simulink model "ZynqBF_2tx_fpga"  (R2018b)
settings: Solver=FixedStepDiscrete  StartTime=0.0  StopTime=10.0  FixedStep=(1/420e3)/128  RelTol=1e-3
undefined symbols (not defined in the file): a, b, c, gs1_i, gs1_q, gs2_i, gs2_q, gs_length
libraries: hdlsllib x65, simulink x41
(part 3 of 4)

== system ZynqBF_2tx_fpga/channel_estimator/peakdetect_ch1/correlator1/sum_elements_i ==
  din : Inport  Partition=on  PartitionDimension=1  PartitionWidth=8  PartitionOffset=0
  start : Inport  Port=2
  Add : Sum  OutDataTypeStr=fixdt(1,32,16)
  Compare To Constant1 : simulink/Logic and Bit Operations/Compare To Constant  relop===  const=7  OutDataTypeStr=boolean
  Compare To Constant2 : simulink/Logic and Bit Operations/Compare To Constant  relop===  const=1  OutDataTypeStr=boolean
  Constant : Constant  Value=0  OutDataTypeStr=fixdt(1,32,16)  SampleTime=-1
  Constant1 : Constant  Value=0  OutDataTypeStr=fixdt(1,16,15)  SampleTime=-1
  Data Type Conversion : DataTypeConversion  OutDataTypeStr=uint8
  Delay1 : Delay  DelayLength=1
  For Each : ForEach  DisableCoverage=on  IndexMode=One-based
  HDL Counter : hdlsllib/Sources/HDL Counter  CountType=Free running  CountInit=0  CountStep=1  CountMax=64  CountFromType=Initial value  CountFrom=0  CountResetPort=on  CountLoadPort=off  CountEnbPort=on  CountDirPort=off  CountDataType=Unsigned  CountWordLen=3  CountFracLen=0  CountSampTime=1
      settings: SourceProductBaseCode=HD
  HDL Counter1 : hdlsllib/Sources/HDL Counter  CountType=Free running  CountInit=0  CountStep=1  CountMax=64  CountFromType=Initial value  CountFrom=0  CountResetPort=off  CountLoadPort=off  CountEnbPort=on  CountDirPort=off  CountDataType=Unsigned  CountWordLen=1  CountFracLen=0  CountSampTime=1
      settings: SourceProductBaseCode=HD
  Logical Operator : Logic  Operator=OR  IconShape=distinctive  AllPortsSameDT=off  OutDataTypeStr=boolean
  Selector : Selector  IndexMode=Zero-based  InputPortWidth=8  IndexOptions=Starting index (port)  Indices=[1 3]  OutputSizes=1
  Switch : Switch  Criteria=u2 ~= 0
  Switch1 : Switch  Criteria=u2 ~= 0
  dout : Outport  ConcatenationDimension=1
  vout : Outport  Port=2  ConcatenationDimension=1
  wires:
  start/1 -> Logical Operator/1, Switch/2, HDL Counter/1
  Add/1 -> Delay1/1, dout/1
  Compare To Constant2/1 -> Switch1/2, HDL Counter/2
  Compare To Constant1/1 -> Logical Operator/2, vout/1
  Delay1/1 -> Switch/3
  Switch/1 -> Add/2
  Constant/1 -> Switch/1
  Switch1/1 -> Add/1
  Constant1/1 -> Switch1/3
  HDL Counter1/1 -> Compare To Constant2/1
  Selector/1 -> Switch1/1
  din/1 -> Selector/1
  Data Type Conversion/1 -> Selector/2
  Logical Operator/1 -> HDL Counter1/1
  HDL Counter/1 -> Compare To Constant1/1, Data Type Conversion/1

== system ZynqBF_2tx_fpga/channel_estimator/peakdetect_ch1/correlator1/sum_elements_q ==
  din : Inport  Partition=on  PartitionDimension=1  PartitionWidth=8  PartitionOffset=0
  start : Inport  Port=2
  Add : Sum  OutDataTypeStr=fixdt(1,32,16)
  Compare To Constant1 : simulink/Logic and Bit Operations/Compare To Constant  relop===  const=7  OutDataTypeStr=boolean
  Compare To Constant2 : simulink/Logic and Bit Operations/Compare To Constant  relop===  const=1  OutDataTypeStr=boolean
  Constant : Constant  Value=0  OutDataTypeStr=fixdt(1,32,16)  SampleTime=-1
  Constant1 : Constant  Value=0  OutDataTypeStr=fixdt(1,16,15)  SampleTime=-1
  Data Type Conversion : DataTypeConversion  OutDataTypeStr=uint8
  Delay1 : Delay  DelayLength=1
  For Each : ForEach  DisableCoverage=on  IndexMode=One-based
  HDL Counter : hdlsllib/Sources/HDL Counter  CountType=Free running  CountInit=0  CountStep=1  CountMax=64  CountFromType=Initial value  CountFrom=0  CountResetPort=on  CountLoadPort=off  CountEnbPort=on  CountDirPort=off  CountDataType=Unsigned  CountWordLen=3  CountFracLen=0  CountSampTime=1
      settings: SourceProductBaseCode=HD
  HDL Counter1 : hdlsllib/Sources/HDL Counter  CountType=Free running  CountInit=0  CountStep=1  CountMax=64  CountFromType=Initial value  CountFrom=0  CountResetPort=off  CountLoadPort=off  CountEnbPort=on  CountDirPort=off  CountDataType=Unsigned  CountWordLen=1  CountFracLen=0  CountSampTime=1
      settings: SourceProductBaseCode=HD
  Logical Operator : Logic  Operator=OR  IconShape=distinctive  AllPortsSameDT=off  OutDataTypeStr=boolean
  Selector : Selector  IndexMode=Zero-based  InputPortWidth=8  IndexOptions=Starting index (port)  Indices=[1 3]  OutputSizes=1
  Switch : Switch  Criteria=u2 ~= 0
  Switch1 : Switch  Criteria=u2 ~= 0
  dout : Outport  ConcatenationDimension=1
  vout : Outport  Port=2  ConcatenationDimension=1
  wires:
  start/1 -> Logical Operator/1, Switch/2, HDL Counter/1
  Add/1 -> Delay1/1, dout/1
  Compare To Constant2/1 -> Switch1/2, HDL Counter/2
  Compare To Constant1/1 -> Logical Operator/2, vout/1
  Delay1/1 -> Switch/3
  Switch/1 -> Add/2
  Constant/1 -> Switch/1
  Switch1/1 -> Add/1
  Constant1/1 -> Switch1/3
  HDL Counter1/1 -> Compare To Constant2/1
  Selector/1 -> Switch1/1
  din/1 -> Selector/1
  Data Type Conversion/1 -> Selector/2
  Logical Operator/1 -> HDL Counter1/1
  HDL Counter/1 -> Compare To Constant1/1, Data Type Conversion/1

== system ZynqBF_2tx_fpga/channel_estimator/peakdetect_ch2/correlator2/correlation_config ==
  rst : Inport
  vin : Inport  Port=2
  Bit Slice : hdlsllib/Logic and Bit Operations/Bit Slice  lidx=14  ridx=6
  Delay{1..2,4..5} (4 alike) : Delay  DelayLength=1
  Delay6 : Delay  DelayLength=3
  correlation_count : hdlsllib/Sources/HDL Counter  CountType=Free running  CountInit=2^15 - 1  CountStep=1  CountMax=25  CountFromType=Initial value  CountFrom=2^15 - 1  CountResetPort=on  CountLoadPort=off  CountEnbPort=on  CountDirPort=off  CountDataType=Unsigned  CountWordLen=15  CountFracLen=0  CountSampTime=1
      settings: SourceProductBaseCode=HD
  shift_count : hdlsllib/Sources/HDL Counter  CountType=Free running  CountInit=63  CountStep=1  CountMax=1  CountFromType=Initial value  CountFrom=63  CountResetPort=on  CountLoadPort=off  CountEnbPort=on  CountDirPort=off  CountDataType=Unsigned  CountWordLen=6  CountFracLen=0  CountSampTime=1
      settings: SourceProductBaseCode=HD
  addr : Outport
  shift : Outport  Port=2
  vout : Outport  Port=3
  wires:
  Delay6/1 -> vout/1
  shift_count/1 -> Delay5/1
  Delay5/1 -> shift/1
  Delay4/1 -> correlation_count/1, shift_count/1
  Delay2/1 -> addr/1
  Delay1/1 -> correlation_count/2, shift_count/2, Delay6/1
  rst/1 -> Delay4/1
  Bit Slice/1 -> Delay2/1
  vin/1 -> Delay1/1
  correlation_count/1 -> Bit Slice/1

== system ZynqBF_2tx_fpga/channel_estimator/peakdetect_ch2/correlator2/correlator_en ==
  valid : Inport
  done : Inport  Port=2
  addri : Inport  Port=3
  Compare To Constant : simulink/Logic and Bit Operations/Compare To Constant  relop===  const=1  OutDataTypeStr=boolean
  Delay1 : Delay  DelayLength=1
  Delay2 : Delay  DelayLength=1
  Delay3 : Delay  DelayLength=1
  Sum : Sum  Inputs=|++
  corr_addr : hdlsllib/Sources/HDL Counter  CountType=Count limited  CountInit=0  CountStep=1  CountMax=63  CountFromType=Initial value  CountFrom=0  CountResetPort=on  CountLoadPort=off  CountEnbPort=on  CountDirPort=off  CountDataType=Unsigned  CountWordLen=6  CountFracLen=0  CountSampTime=1
      settings: SourceProductBaseCode=HD
  corr_state : hdlsllib/Sources/HDL Counter  CountType=Count limited  CountInit=0  CountStep=1  CountMax=1  CountFromType=Initial value  CountFrom=0  CountResetPort=on  CountLoadPort=off  CountEnbPort=on  CountDirPort=off  CountDataType=Unsigned  CountWordLen=6  CountFracLen=0  CountSampTime=1
      settings: SourceProductBaseCode=HD
  start : Outport
  en : Outport  Port=2
  gs_addr : Outport  Port=3
  rx_addr : Outport  Port=4
  wires:
  addri/1 -> Sum/2
  Sum/1 -> rx_addr/1
  corr_addr/1 -> Sum/1, gs_addr/1
  Delay3/1 -> start/1
  Delay2/1 -> en/1, corr_addr/2
  Delay1/1 -> Delay3/1, corr_state/2
  done/1 -> corr_state/1
  Compare To Constant/1 -> Delay2/1
  corr_state/1 -> Compare To Constant/1
  valid/1 -> Delay1/1, corr_addr/1

== system ZynqBF_2tx_fpga/channel_estimator/peakdetect_ch2/correlator2/correlator_i ==
  rx : Inport  Partition=on  PartitionDimension=1  PartitionWidth=1  PartitionOffset=0
  gs : Inport  Port=2  Partition=on  PartitionDimension=1  PartitionWidth=1  PartitionOffset=0
  start : Inport  Port=3
  vin : Inport  Port=4
  Compare To Constant1 : simulink/Logic and Bit Operations/Compare To Constant  relop===  const=63  OutDataTypeStr=boolean
  Constant : Constant  Value=0  OutDataTypeStr=fixdt(1,32,16)  SampleTime=-1
  Constant1 : Constant  Value=0  OutDataTypeStr=fixdt(1,16,15)  SampleTime=-1
  Delay1 : Delay  DelayLength=1
  For Each : ForEach  DisableCoverage=on  IndexMode=One-based
  HDL Counter : hdlsllib/Sources/HDL Counter  CountType=Free running  CountInit=0  CountStep=1  CountMax=64  CountFromType=Initial value  CountFrom=0  CountResetPort=on  CountLoadPort=off  CountEnbPort=on  CountDirPort=off  CountDataType=Unsigned  CountWordLen=7  CountFracLen=0  CountSampTime=1
      settings: SourceProductBaseCode=HD
  Multiply-Add : hdlsllib/HDL Operations/Multiply-Add  Function=c+(a.*b)  datatype=fixdt(1,32,16)  DoSatur=off  FMA=off
      settings: SourceProductName=HDL Coder  SourceProductBaseCode=HD
  Switch : Switch  Criteria=u2 ~= 0
  Switch1 : Switch  Criteria=u2 ~= 0
  Switch2 : Switch  Criteria=u2 ~= 0
  correlator_mac : hdlsllib/HDL Operations/Multiply-Accumulate  Commented=on  opMode=Streaming - using Start and End ports  initValueSetting=Dialog  initValue=0  initValueSetting2=Dialog  initValue2=0  initValueSetting3=Dialog  initValue3=0  num_samples=2  RndMeth2=Floor  RndMeth3=Floor  datatype2=Inherit: Inherit via back propagation  datatype3=Inherit: Inherit via back propagation  validOut=off  endInandOut=on  startOut=off  countOut=on  dim=-1  DoSatur=off  parallel=off
      settings: SourceProductName=HDL Coder  SourceProductBaseCode=HD
  dout : Outport  ConcatenationDimension=1
  vout : Outport  Port=2  ConcatenationDimension=1
  wires:
  Constant1/1 -> Switch2/3, Switch1/3
  Switch2/1 -> Multiply-Add/2
  Switch1/1 -> Multiply-Add/1
  Constant/1 -> Switch/1
  Switch/1 -> Multiply-Add/3
  Delay1/1 -> Switch/3
  gs/1 -> Switch2/1
  Compare To Constant1/1 -> vout/1
  HDL Counter/1 -> Compare To Constant1/1
  vin/1 -> HDL Counter/2, Switch2/2, Switch1/2
  Multiply-Add/1 -> dout/1, Delay1/1
  start/1 -> HDL Counter/1, Switch/2
  rx/1 -> Switch1/1

== system ZynqBF_2tx_fpga/channel_estimator/peakdetect_ch2/correlator2/correlator_q ==
  rx : Inport  Partition=on  PartitionDimension=1  PartitionWidth=1  PartitionOffset=0
  gs : Inport  Port=2  Partition=on  PartitionDimension=1  PartitionWidth=1  PartitionOffset=0
  start : Inport  Port=3
  vin : Inport  Port=4
  Compare To Constant1 : simulink/Logic and Bit Operations/Compare To Constant  relop===  const=63  OutDataTypeStr=boolean
  Constant : Constant  Value=0  OutDataTypeStr=fixdt(1,32,16)  SampleTime=-1
  Constant1 : Constant  Value=0  OutDataTypeStr=fixdt(1,16,15)  SampleTime=-1
  Delay1 : Delay  DelayLength=1
  For Each : ForEach  DisableCoverage=on  IndexMode=One-based
  HDL Counter : hdlsllib/Sources/HDL Counter  CountType=Free running  CountInit=0  CountStep=1  CountMax=64  CountFromType=Initial value  CountFrom=0  CountResetPort=on  CountLoadPort=off  CountEnbPort=on  CountDirPort=off  CountDataType=Unsigned  CountWordLen=7  CountFracLen=0  CountSampTime=1
      settings: SourceProductBaseCode=HD
  Multiply-Add : hdlsllib/HDL Operations/Multiply-Add  Function=c+(a.*b)  datatype=fixdt(1,32,16)  DoSatur=off  FMA=off
      settings: SourceProductName=HDL Coder  SourceProductBaseCode=HD
  Switch : Switch  Criteria=u2 ~= 0
  Switch1 : Switch  Criteria=u2 ~= 0
  Switch2 : Switch  Criteria=u2 ~= 0
  correlator_mac : hdlsllib/HDL Operations/Multiply-Accumulate  Commented=on  opMode=Streaming - using Start and End ports  initValueSetting=Dialog  initValue=0  initValueSetting2=Dialog  initValue2=0  initValueSetting3=Dialog  initValue3=0  num_samples=2  RndMeth2=Floor  RndMeth3=Floor  datatype2=Inherit: Inherit via back propagation  datatype3=Inherit: Inherit via back propagation  validOut=off  endInandOut=on  startOut=off  countOut=on  dim=-1  DoSatur=off  parallel=off
      settings: SourceProductName=HDL Coder  SourceProductBaseCode=HD
  dout : Outport  ConcatenationDimension=1
  vout : Outport  Port=2  ConcatenationDimension=1
  wires:
  Constant1/1 -> Switch2/3, Switch1/3
  Switch2/1 -> Multiply-Add/2
  Switch1/1 -> Multiply-Add/1
  Constant/1 -> Switch/1
  Switch/1 -> Multiply-Add/3
  Delay1/1 -> Switch/3
  gs/1 -> Switch2/1
  Compare To Constant1/1 -> vout/1
  HDL Counter/1 -> Compare To Constant1/1
  vin/1 -> HDL Counter/2, Switch2/2, Switch1/2
  Multiply-Add/1 -> dout/1, Delay1/1
  start/1 -> HDL Counter/1, Switch/2
  rx/1 -> Switch1/1

== system ZynqBF_2tx_fpga/channel_estimator/peakdetect_ch2/correlator2/data_in ==
  rst : Inport
  valid : Inport  Port=2
  Bit Rotate : hdlsllib/Logic and Bit Operations/Bit Rotate  mode=Rotate Left  N=1
      settings: SourceProductName=HDL Coder  SourceProductBaseCode=HD
  Compare To Constant : simulink/Logic and Bit Operations/Compare To Constant  relop===  const=63  OutDataTypeStr=boolean
  Constant1 : Constant  Value=0  OutDataTypeStr=fixdt(0,64,0)  SampleTime=-1
  Delay{,2..4,6} (5 alike) : Delay  DelayLength=1
  Delay1 : Delay  DelayLength=1  InitialCondition=(2^63)
  Delay5 : Delay  DelayLength=3
  Logical Operator : Logic  IconShape=distinctive  AllPortsSameDT=off  OutDataTypeStr=boolean
  Switch1 : Switch  Criteria=u2 ~= 0
  Switch2 : Switch  Criteria=u2 ~= 0
  addr_counter : hdlsllib/Sources/HDL Counter  CountType=Count limited  CountInit=63  CountStep=1  CountMax=511  CountFromType=Initial value  CountFrom=63  CountResetPort=on  CountLoadPort=off  CountEnbPort=on  CountDirPort=off  CountDataType=Unsigned  CountWordLen=9  CountFracLen=0  CountSampTime=1
      settings: SourceProductBaseCode=HD
  ram_counter : hdlsllib/Sources/HDL Counter  CountType=Free running  CountInit=63  CountStep=1  CountMax=63  CountFromType=Initial value  CountFrom=63  CountResetPort=on  CountLoadPort=off  CountEnbPort=on  CountDirPort=off  CountDataType=Unsigned  CountWordLen=6  CountFracLen=0  CountSampTime=1
      settings: SourceProductBaseCode=HD
  addr : Outport
  we : Outport  Port=2
  wires:
  Delay5/1 -> addr/1
  Delay6/1 -> Delay/1, Switch1/2
  Delay4/1 -> addr_counter/1, ram_counter/1  "rst"
  Delay3/1 -> ram_counter/2, Logical Operator/2, Delay6/1
  Delay2/1 -> we/1
  Switch2/1 -> Delay2/1
  Delay/1 -> Switch2/2
  Constant1/1 -> Switch2/3
  Bit Rotate/1 -> Switch1/1
  Switch1/1 -> Switch2/1, Delay1/1
  Delay1/1 -> Bit Rotate/1, Switch1/3
  Compare To Constant/1 -> Logical Operator/1
  Logical Operator/1 -> addr_counter/2
  rst/1 -> Delay4/1
  ram_counter/1 -> Compare To Constant/1
  valid/1 -> Delay3/1
  addr_counter/1 -> Delay5/1

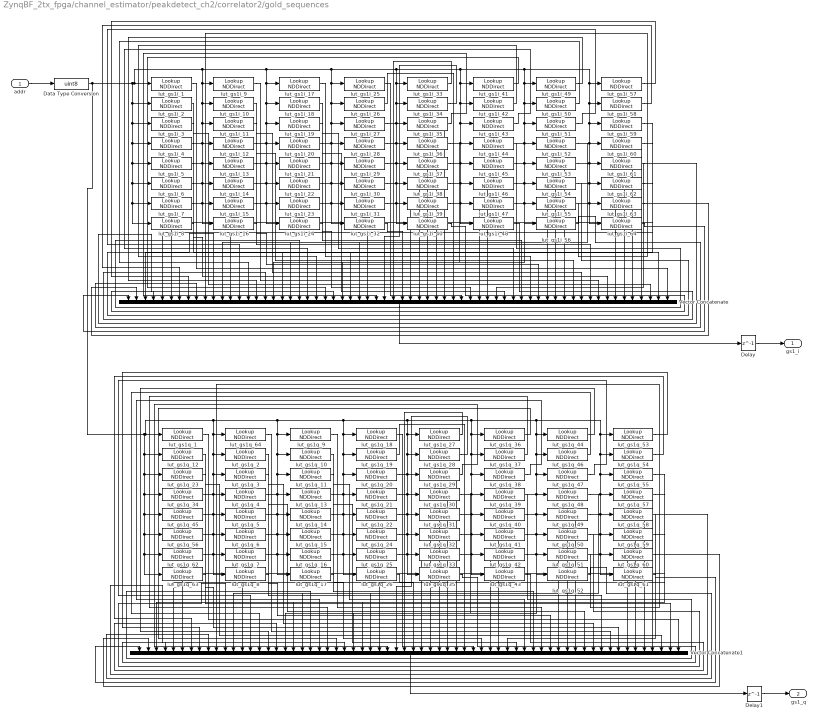
== system ZynqBF_2tx_fpga/channel_estimator/peakdetect_ch2/correlator2/gold_sequences ==
  addr : Inport
  Data Type Conversion : DataTypeConversion  OutDataTypeStr=uint8
  Delay : Delay  DelayLength=1
  Delay1 : Delay  DelayLength=1
  Vector Concatenate : Concatenate  NumInputs=64
  Vector Concatenate1 : Concatenate  NumInputs=64
  lut_gs1i_1 : LookupNDDirect  NumberOfTableDimensions=1  Table=gs2_i_f(1:64:end)  DiagnosticForOutOfRangeInput=Error  TableDataTypeStr=fixdt(1,16,15)
  lut_gs1i_10 : LookupNDDirect  NumberOfTableDimensions=1  Table=gs2_i_f(10:64:end)  DiagnosticForOutOfRangeInput=Error  TableDataTypeStr=fixdt(1,16,15)
  lut_gs1i_11 : LookupNDDirect  NumberOfTableDimensions=1  Table=gs2_i_f(11:64:end)  DiagnosticForOutOfRangeInput=Error  TableDataTypeStr=fixdt(1,16,15)
  lut_gs1i_12 : LookupNDDirect  NumberOfTableDimensions=1  Table=gs2_i_f(12:64:end)  DiagnosticForOutOfRangeInput=Error  TableDataTypeStr=fixdt(1,16,15)
  lut_gs1i_13 : LookupNDDirect  NumberOfTableDimensions=1  Table=gs2_i_f(13:64:end)  DiagnosticForOutOfRangeInput=Error  TableDataTypeStr=fixdt(1,16,15)
  lut_gs1i_14 : LookupNDDirect  NumberOfTableDimensions=1  Table=gs2_i_f(14:64:end)  DiagnosticForOutOfRangeInput=Error  TableDataTypeStr=fixdt(1,16,15)
  lut_gs1i_15 : LookupNDDirect  NumberOfTableDimensions=1  Table=gs2_i_f(15:64:end)  DiagnosticForOutOfRangeInput=Error  TableDataTypeStr=fixdt(1,16,15)
  lut_gs1i_16 : LookupNDDirect  NumberOfTableDimensions=1  Table=gs2_i_f(16:64:end)  DiagnosticForOutOfRangeInput=Error  TableDataTypeStr=fixdt(1,16,15)
  lut_gs1i_17 : LookupNDDirect  NumberOfTableDimensions=1  Table=gs2_i_f(17:64:end)  DiagnosticForOutOfRangeInput=Error  TableDataTypeStr=fixdt(1,16,15)
  lut_gs1i_18 : LookupNDDirect  NumberOfTableDimensions=1  Table=gs2_i_f(18:64:end)  DiagnosticForOutOfRangeInput=Error  TableDataTypeStr=fixdt(1,16,15)
  lut_gs1i_19 : LookupNDDirect  NumberOfTableDimensions=1  Table=gs2_i_f(19:64:end)  DiagnosticForOutOfRangeInput=Error  TableDataTypeStr=fixdt(1,16,15)
  lut_gs1i_2 : LookupNDDirect  NumberOfTableDimensions=1  Table=gs2_i_f(2:64:end)  DiagnosticForOutOfRangeInput=Error  TableDataTypeStr=fixdt(1,16,15)
  lut_gs1i_20 : LookupNDDirect  NumberOfTableDimensions=1  Table=gs2_i_f(20:64:end)  DiagnosticForOutOfRangeInput=Error  TableDataTypeStr=fixdt(1,16,15)
  lut_gs1i_21 : LookupNDDirect  NumberOfTableDimensions=1  Table=gs2_i_f(21:64:end)  DiagnosticForOutOfRangeInput=Error  TableDataTypeStr=fixdt(1,16,15)
  lut_gs1i_22 : LookupNDDirect  NumberOfTableDimensions=1  Table=gs2_i_f(22:64:end)  DiagnosticForOutOfRangeInput=Error  TableDataTypeStr=fixdt(1,16,15)
  lut_gs1i_23 : LookupNDDirect  NumberOfTableDimensions=1  Table=gs2_i_f(23:64:end)  DiagnosticForOutOfRangeInput=Error  TableDataTypeStr=fixdt(1,16,15)
  lut_gs1i_24 : LookupNDDirect  NumberOfTableDimensions=1  Table=gs2_i_f(24:64:end)  DiagnosticForOutOfRangeInput=Error  TableDataTypeStr=fixdt(1,16,15)
  lut_gs1i_25 : LookupNDDirect  NumberOfTableDimensions=1  Table=gs2_i_f(25:64:end)  DiagnosticForOutOfRangeInput=Error  TableDataTypeStr=fixdt(1,16,15)
  lut_gs1i_26 : LookupNDDirect  NumberOfTableDimensions=1  Table=gs2_i_f(26:64:end)  DiagnosticForOutOfRangeInput=Error  TableDataTypeStr=fixdt(1,16,15)
  lut_gs1i_27 : LookupNDDirect  NumberOfTableDimensions=1  Table=gs2_i_f(27:64:end)  DiagnosticForOutOfRangeInput=Error  TableDataTypeStr=fixdt(1,16,15)
  lut_gs1i_28 : LookupNDDirect  NumberOfTableDimensions=1  Table=gs2_i_f(28:64:end)  DiagnosticForOutOfRangeInput=Error  TableDataTypeStr=fixdt(1,16,15)
  lut_gs1i_29 : LookupNDDirect  NumberOfTableDimensions=1  Table=gs2_i_f(29:64:end)  DiagnosticForOutOfRangeInput=Error  TableDataTypeStr=fixdt(1,16,15)
  lut_gs1i_3 : LookupNDDirect  NumberOfTableDimensions=1  Table=gs2_i_f(3:64:end)  DiagnosticForOutOfRangeInput=Error  TableDataTypeStr=fixdt(1,16,15)
  lut_gs1i_30 : LookupNDDirect  NumberOfTableDimensions=1  Table=gs2_i_f(30:64:end)  DiagnosticForOutOfRangeInput=Error  TableDataTypeStr=fixdt(1,16,15)
  lut_gs1i_31 : LookupNDDirect  NumberOfTableDimensions=1  Table=gs2_i_f(31:64:end)  DiagnosticForOutOfRangeInput=Error  TableDataTypeStr=fixdt(1,16,15)
  lut_gs1i_32 : LookupNDDirect  NumberOfTableDimensions=1  Table=gs2_i_f(32:64:end)  DiagnosticForOutOfRangeInput=Error  TableDataTypeStr=fixdt(1,16,15)
  lut_gs1i_33 : LookupNDDirect  NumberOfTableDimensions=1  Table=gs2_i_f(33:64:end)  DiagnosticForOutOfRangeInput=Error  TableDataTypeStr=fixdt(1,16,15)
  lut_gs1i_34 : LookupNDDirect  NumberOfTableDimensions=1  Table=gs2_i_f(34:64:end)  DiagnosticForOutOfRangeInput=Error  TableDataTypeStr=fixdt(1,16,15)
  lut_gs1i_35 : LookupNDDirect  NumberOfTableDimensions=1  Table=gs2_i_f(35:64:end)  DiagnosticForOutOfRangeInput=Error  TableDataTypeStr=fixdt(1,16,15)
  lut_gs1i_36 : LookupNDDirect  NumberOfTableDimensions=1  Table=gs2_i_f(36:64:end)  DiagnosticForOutOfRangeInput=Error  TableDataTypeStr=fixdt(1,16,15)
  lut_gs1i_37 : LookupNDDirect  NumberOfTableDimensions=1  Table=gs2_i_f(37:64:end)  DiagnosticForOutOfRangeInput=Error  TableDataTypeStr=fixdt(1,16,15)
  lut_gs1i_38 : LookupNDDirect  NumberOfTableDimensions=1  Table=gs2_i_f(38:64:end)  DiagnosticForOutOfRangeInput=Error  TableDataTypeStr=fixdt(1,16,15)
  lut_gs1i_39 : LookupNDDirect  NumberOfTableDimensions=1  Table=gs2_i_f(39:64:end)  DiagnosticForOutOfRangeInput=Error  TableDataTypeStr=fixdt(1,16,15)
  lut_gs1i_4 : LookupNDDirect  NumberOfTableDimensions=1  Table=gs2_i_f(4:64:end)  DiagnosticForOutOfRangeInput=Error  TableDataTypeStr=fixdt(1,16,15)
  lut_gs1i_40 : LookupNDDirect  NumberOfTableDimensions=1  Table=gs2_i_f(40:64:end)  DiagnosticForOutOfRangeInput=Error  TableDataTypeStr=fixdt(1,16,15)
  lut_gs1i_41 : LookupNDDirect  NumberOfTableDimensions=1  Table=gs2_i_f(41:64:end)  DiagnosticForOutOfRangeInput=Error  TableDataTypeStr=fixdt(1,16,15)
  lut_gs1i_42 : LookupNDDirect  NumberOfTableDimensions=1  Table=gs2_i_f(42:64:end)  DiagnosticForOutOfRangeInput=Error  TableDataTypeStr=fixdt(1,16,15)
  lut_gs1i_43 : LookupNDDirect  NumberOfTableDimensions=1  Table=gs2_i_f(43:64:end)  DiagnosticForOutOfRangeInput=Error  TableDataTypeStr=fixdt(1,16,15)
  lut_gs1i_44 : LookupNDDirect  NumberOfTableDimensions=1  Table=gs2_i_f(44:64:end)  DiagnosticForOutOfRangeInput=Error  TableDataTypeStr=fixdt(1,16,15)
  lut_gs1i_45 : LookupNDDirect  NumberOfTableDimensions=1  Table=gs2_i_f(45:64:end)  DiagnosticForOutOfRangeInput=Error  TableDataTypeStr=fixdt(1,16,15)
  lut_gs1i_46 : LookupNDDirect  NumberOfTableDimensions=1  Table=gs2_i_f(46:64:end)  DiagnosticForOutOfRangeInput=Error  TableDataTypeStr=fixdt(1,16,15)
  lut_gs1i_47 : LookupNDDirect  NumberOfTableDimensions=1  Table=gs2_i_f(47:64:end)  DiagnosticForOutOfRangeInput=Error  TableDataTypeStr=fixdt(1,16,15)
  lut_gs1i_48 : LookupNDDirect  NumberOfTableDimensions=1  Table=gs2_i_f(48:64:end)  DiagnosticForOutOfRangeInput=Error  TableDataTypeStr=fixdt(1,16,15)
  lut_gs1i_49 : LookupNDDirect  NumberOfTableDimensions=1  Table=gs2_i_f(49:64:end)  DiagnosticForOutOfRangeInput=Error  TableDataTypeStr=fixdt(1,16,15)
  lut_gs1i_5 : LookupNDDirect  NumberOfTableDimensions=1  Table=gs2_i_f(5:64:end)  DiagnosticForOutOfRangeInput=Error  TableDataTypeStr=fixdt(1,16,15)
  lut_gs1i_50 : LookupNDDirect  NumberOfTableDimensions=1  Table=gs2_i_f(50:64:end)  DiagnosticForOutOfRangeInput=Error  TableDataTypeStr=fixdt(1,16,15)
  lut_gs1i_51 : LookupNDDirect  NumberOfTableDimensions=1  Table=gs2_i_f(51:64:end)  DiagnosticForOutOfRangeInput=Error  TableDataTypeStr=fixdt(1,16,15)
  lut_gs1i_52 : LookupNDDirect  NumberOfTableDimensions=1  Table=gs2_i_f(52:64:end)  DiagnosticForOutOfRangeInput=Error  TableDataTypeStr=fixdt(1,16,15)
  lut_gs1i_53 : LookupNDDirect  NumberOfTableDimensions=1  Table=gs2_i_f(53:64:end)  DiagnosticForOutOfRangeInput=Error  TableDataTypeStr=fixdt(1,16,15)
  lut_gs1i_54 : LookupNDDirect  NumberOfTableDimensions=1  Table=gs2_i_f(54:64:end)  DiagnosticForOutOfRangeInput=Error  TableDataTypeStr=fixdt(1,16,15)
  lut_gs1i_55 : LookupNDDirect  NumberOfTableDimensions=1  Table=gs2_i_f(55:64:end)  DiagnosticForOutOfRangeInput=Error  TableDataTypeStr=fixdt(1,16,15)
  lut_gs1i_56 : LookupNDDirect  NumberOfTableDimensions=1  Table=gs2_i_f(56:64:end)  DiagnosticForOutOfRangeInput=Error  TableDataTypeStr=fixdt(1,16,15)
  lut_gs1i_57 : LookupNDDirect  NumberOfTableDimensions=1  Table=gs2_i_f(57:64:end)  DiagnosticForOutOfRangeInput=Error  TableDataTypeStr=fixdt(1,16,15)
  lut_gs1i_58 : LookupNDDirect  NumberOfTableDimensions=1  Table=gs2_i_f(58:64:end)  DiagnosticForOutOfRangeInput=Error  TableDataTypeStr=fixdt(1,16,15)
  lut_gs1i_59 : LookupNDDirect  NumberOfTableDimensions=1  Table=gs2_i_f(59:64:end)  DiagnosticForOutOfRangeInput=Error  TableDataTypeStr=fixdt(1,16,15)
  lut_gs1i_6 : LookupNDDirect  NumberOfTableDimensions=1  Table=gs2_i_f(6:64:end)  DiagnosticForOutOfRangeInput=Error  TableDataTypeStr=fixdt(1,16,15)
  lut_gs1i_60 : LookupNDDirect  NumberOfTableDimensions=1  Table=gs2_i_f(60:64:end)  DiagnosticForOutOfRangeInput=Error  TableDataTypeStr=fixdt(1,16,15)
  lut_gs1i_61 : LookupNDDirect  NumberOfTableDimensions=1  Table=gs2_i_f(61:64:end)  DiagnosticForOutOfRangeInput=Error  TableDataTypeStr=fixdt(1,16,15)
  lut_gs1i_62 : LookupNDDirect  NumberOfTableDimensions=1  Table=gs2_i_f(62:64:end)  DiagnosticForOutOfRangeInput=Error  TableDataTypeStr=fixdt(1,16,15)
  lut_gs1i_63 : LookupNDDirect  NumberOfTableDimensions=1  Table=gs2_i_f(63:64:end)  DiagnosticForOutOfRangeInput=Error  TableDataTypeStr=fixdt(1,16,15)
  lut_gs1i_64 : LookupNDDirect  NumberOfTableDimensions=1  Table=gs2_i_f(64:64:end)  DiagnosticForOutOfRangeInput=Error  TableDataTypeStr=fixdt(1,16,15)
  lut_gs1i_7 : LookupNDDirect  NumberOfTableDimensions=1  Table=gs2_i_f(7:64:end)  DiagnosticForOutOfRangeInput=Error  TableDataTypeStr=fixdt(1,16,15)
  lut_gs1i_8 : LookupNDDirect  NumberOfTableDimensions=1  Table=gs2_i_f(8:64:end)  DiagnosticForOutOfRangeInput=Error  TableDataTypeStr=fixdt(1,16,15)
  lut_gs1i_9 : LookupNDDirect  NumberOfTableDimensions=1  Table=gs2_i_f(9:64:end)  DiagnosticForOutOfRangeInput=Error  TableDataTypeStr=fixdt(1,16,15)
  lut_gs1q_1 : LookupNDDirect  NumberOfTableDimensions=1  Table=gs2_q_f(1:64:end)  DiagnosticForOutOfRangeInput=Error  TableDataTypeStr=fixdt(1,16,15)
  lut_gs1q_10 : LookupNDDirect  NumberOfTableDimensions=1  Table=gs2_q_f(18:64:end)  DiagnosticForOutOfRangeInput=Error  TableDataTypeStr=fixdt(1,16,15)
  lut_gs1q_11 : LookupNDDirect  NumberOfTableDimensions=1  Table=gs2_q_f(19:64:end)  DiagnosticForOutOfRangeInput=Error  TableDataTypeStr=fixdt(1,16,15)
  lut_gs1q_12 : LookupNDDirect  NumberOfTableDimensions=1  Table=gs2_q_f(2:64:end)  DiagnosticForOutOfRangeInput=Error  TableDataTypeStr=fixdt(1,16,15)
  lut_gs1q_13 : LookupNDDirect  NumberOfTableDimensions=1  Table=gs2_q_f(20:64:end)  DiagnosticForOutOfRangeInput=Error  TableDataTypeStr=fixdt(1,16,15)
  lut_gs1q_14 : LookupNDDirect  NumberOfTableDimensions=1  Table=gs2_q_f(21:64:end)  DiagnosticForOutOfRangeInput=Error  TableDataTypeStr=fixdt(1,16,15)
  lut_gs1q_15 : LookupNDDirect  NumberOfTableDimensions=1  Table=gs2_q_f(22:64:end)  DiagnosticForOutOfRangeInput=Error  TableDataTypeStr=fixdt(1,16,15)
  lut_gs1q_16 : LookupNDDirect  NumberOfTableDimensions=1  Table=gs2_q_f(23:64:end)  DiagnosticForOutOfRangeInput=Error  TableDataTypeStr=fixdt(1,16,15)
  lut_gs1q_17 : LookupNDDirect  NumberOfTableDimensions=1  Table=gs2_q_f(24:64:end)  DiagnosticForOutOfRangeInput=Error  TableDataTypeStr=fixdt(1,16,15)
  lut_gs1q_18 : LookupNDDirect  NumberOfTableDimensions=1  Table=gs2_q_f(25:64:end)  DiagnosticForOutOfRangeInput=Error  TableDataTypeStr=fixdt(1,16,15)
  lut_gs1q_19 : LookupNDDirect  NumberOfTableDimensions=1  Table=gs2_q_f(26:64:end)  DiagnosticForOutOfRangeInput=Error  TableDataTypeStr=fixdt(1,16,15)
  lut_gs1q_2 : LookupNDDirect  NumberOfTableDimensions=1  Table=gs2_q_f(10:64:end)  DiagnosticForOutOfRangeInput=Error  TableDataTypeStr=fixdt(1,16,15)
  lut_gs1q_20 : LookupNDDirect  NumberOfTableDimensions=1  Table=gs2_q_f(27:64:end)  DiagnosticForOutOfRangeInput=Error  TableDataTypeStr=fixdt(1,16,15)
  lut_gs1q_21 : LookupNDDirect  NumberOfTableDimensions=1  Table=gs2_q_f(28:64:end)  DiagnosticForOutOfRangeInput=Error  TableDataTypeStr=fixdt(1,16,15)
  lut_gs1q_22 : LookupNDDirect  NumberOfTableDimensions=1  Table=gs2_q_f(29:64:end)  DiagnosticForOutOfRangeInput=Error  TableDataTypeStr=fixdt(1,16,15)
  lut_gs1q_23 : LookupNDDirect  NumberOfTableDimensions=1  Table=gs2_q_f(3:64:end)  DiagnosticForOutOfRangeInput=Error  TableDataTypeStr=fixdt(1,16,15)
  lut_gs1q_24 : LookupNDDirect  NumberOfTableDimensions=1  Table=gs2_q_f(30:64:end)  DiagnosticForOutOfRangeInput=Error  TableDataTypeStr=fixdt(1,16,15)
  lut_gs1q_25 : LookupNDDirect  NumberOfTableDimensions=1  Table=gs2_q_f(31:64:end)  DiagnosticForOutOfRangeInput=Error  TableDataTypeStr=fixdt(1,16,15)
  lut_gs1q_26 : LookupNDDirect  NumberOfTableDimensions=1  Table=gs2_q_f(32:64:end)  DiagnosticForOutOfRangeInput=Error  TableDataTypeStr=fixdt(1,16,15)
  lut_gs1q_27 : LookupNDDirect  NumberOfTableDimensions=1  Table=gs2_q_f(33:64:end)  DiagnosticForOutOfRangeInput=Error  TableDataTypeStr=fixdt(1,16,15)
  lut_gs1q_28 : LookupNDDirect  NumberOfTableDimensions=1  Table=gs2_q_f(34:64:end)  DiagnosticForOutOfRangeInput=Error  TableDataTypeStr=fixdt(1,16,15)
  lut_gs1q_29 : LookupNDDirect  NumberOfTableDimensions=1  Table=gs2_q_f(35:64:end)  DiagnosticForOutOfRangeInput=Error  TableDataTypeStr=fixdt(1,16,15)
  lut_gs1q_3 : LookupNDDirect  NumberOfTableDimensions=1  Table=gs2_q_f(11:64:end)  DiagnosticForOutOfRangeInput=Error  TableDataTypeStr=fixdt(1,16,15)
  lut_gs1q_30 : LookupNDDirect  NumberOfTableDimensions=1  Table=gs2_q_f(36:64:end)  DiagnosticForOutOfRangeInput=Error  TableDataTypeStr=fixdt(1,16,15)
  lut_gs1q_31 : LookupNDDirect  NumberOfTableDimensions=1  Table=gs2_q_f(37:64:end)  DiagnosticForOutOfRangeInput=Error  TableDataTypeStr=fixdt(1,16,15)
  lut_gs1q_32 : LookupNDDirect  NumberOfTableDimensions=1  Table=gs2_q_f(38:64:end)  DiagnosticForOutOfRangeInput=Error  TableDataTypeStr=fixdt(1,16,15)
  lut_gs1q_33 : LookupNDDirect  NumberOfTableDimensions=1  Table=gs2_q_f(39:64:end)  DiagnosticForOutOfRangeInput=Error  TableDataTypeStr=fixdt(1,16,15)
  lut_gs1q_34 : LookupNDDirect  NumberOfTableDimensions=1  Table=gs2_q_f(4:64:end)  DiagnosticForOutOfRangeInput=Error  TableDataTypeStr=fixdt(1,16,15)
  lut_gs1q_35 : LookupNDDirect  NumberOfTableDimensions=1  Table=gs2_q_f(40:64:end)  DiagnosticForOutOfRangeInput=Error  TableDataTypeStr=fixdt(1,16,15)
  lut_gs1q_36 : LookupNDDirect  NumberOfTableDimensions=1  Table=gs2_q_f(41:64:end)  DiagnosticForOutOfRangeInput=Error  TableDataTypeStr=fixdt(1,16,15)
  lut_gs1q_37 : LookupNDDirect  NumberOfTableDimensions=1  Table=gs2_q_f(42:64:end)  DiagnosticForOutOfRangeInput=Error  TableDataTypeStr=fixdt(1,16,15)
  lut_gs1q_38 : LookupNDDirect  NumberOfTableDimensions=1  Table=gs2_q_f(43:64:end)  DiagnosticForOutOfRangeInput=Error  TableDataTypeStr=fixdt(1,16,15)
  lut_gs1q_39 : LookupNDDirect  NumberOfTableDimensions=1  Table=gs2_q_f(44:64:end)  DiagnosticForOutOfRangeInput=Error  TableDataTypeStr=fixdt(1,16,15)
  lut_gs1q_4 : LookupNDDirect  NumberOfTableDimensions=1  Table=gs2_q_f(12:64:end)  DiagnosticForOutOfRangeInput=Error  TableDataTypeStr=fixdt(1,16,15)
  lut_gs1q_40 : LookupNDDirect  NumberOfTableDimensions=1  Table=gs2_q_f(45:64:end)  DiagnosticForOutOfRangeInput=Error  TableDataTypeStr=fixdt(1,16,15)
  lut_gs1q_41 : LookupNDDirect  NumberOfTableDimensions=1  Table=gs2_q_f(46:64:end)  DiagnosticForOutOfRangeInput=Error  TableDataTypeStr=fixdt(1,16,15)
  lut_gs1q_42 : LookupNDDirect  NumberOfTableDimensions=1  Table=gs2_q_f(47:64:end)  DiagnosticForOutOfRangeInput=Error  TableDataTypeStr=fixdt(1,16,15)
  lut_gs1q_43 : LookupNDDirect  NumberOfTableDimensions=1  Table=gs2_q_f(48:64:end)  DiagnosticForOutOfRangeInput=Error  TableDataTypeStr=fixdt(1,16,15)
  lut_gs1q_44 : LookupNDDirect  NumberOfTableDimensions=1  Table=gs2_q_f(49:64:end)  DiagnosticForOutOfRangeInput=Error  TableDataTypeStr=fixdt(1,16,15)
  lut_gs1q_45 : LookupNDDirect  NumberOfTableDimensions=1  Table=gs2_q_f(5:64:end)  DiagnosticForOutOfRangeInput=Error  TableDataTypeStr=fixdt(1,16,15)
  lut_gs1q_46 : LookupNDDirect  NumberOfTableDimensions=1  Table=gs2_q_f(50:64:end)  DiagnosticForOutOfRangeInput=Error  TableDataTypeStr=fixdt(1,16,15)
  lut_gs1q_47 : LookupNDDirect  NumberOfTableDimensions=1  Table=gs2_q_f(51:64:end)  DiagnosticForOutOfRangeInput=Error  TableDataTypeStr=fixdt(1,16,15)
  lut_gs1q_48 : LookupNDDirect  NumberOfTableDimensions=1  Table=gs2_q_f(52:64:end)  DiagnosticForOutOfRangeInput=Error  TableDataTypeStr=fixdt(1,16,15)
  lut_gs1q_49 : LookupNDDirect  NumberOfTableDimensions=1  Table=gs2_q_f(53:64:end)  DiagnosticForOutOfRangeInput=Error  TableDataTypeStr=fixdt(1,16,15)
  lut_gs1q_5 : LookupNDDirect  NumberOfTableDimensions=1  Table=gs2_q_f(13:64:end)  DiagnosticForOutOfRangeInput=Error  TableDataTypeStr=fixdt(1,16,15)
  lut_gs1q_50 : LookupNDDirect  NumberOfTableDimensions=1  Table=gs2_q_f(54:64:end)  DiagnosticForOutOfRangeInput=Error  TableDataTypeStr=fixdt(1,16,15)
  lut_gs1q_51 : LookupNDDirect  NumberOfTableDimensions=1  Table=gs2_q_f(55:64:end)  DiagnosticForOutOfRangeInput=Error  TableDataTypeStr=fixdt(1,16,15)
  lut_gs1q_52 : LookupNDDirect  NumberOfTableDimensions=1  Table=gs2_q_f(56:64:end)  DiagnosticForOutOfRangeInput=Error  TableDataTypeStr=fixdt(1,16,15)
  lut_gs1q_53 : LookupNDDirect  NumberOfTableDimensions=1  Table=gs2_q_f(57:64:end)  DiagnosticForOutOfRangeInput=Error  TableDataTypeStr=fixdt(1,16,15)
  lut_gs1q_54 : LookupNDDirect  NumberOfTableDimensions=1  Table=gs2_q_f(58:64:end)  DiagnosticForOutOfRangeInput=Error  TableDataTypeStr=fixdt(1,16,15)
  lut_gs1q_55 : LookupNDDirect  NumberOfTableDimensions=1  Table=gs2_q_f(59:64:end)  DiagnosticForOutOfRangeInput=Error  TableDataTypeStr=fixdt(1,16,15)
  lut_gs1q_56 : LookupNDDirect  NumberOfTableDimensions=1  Table=gs2_q_f(6:64:end)  DiagnosticForOutOfRangeInput=Error  TableDataTypeStr=fixdt(1,16,15)
  lut_gs1q_57 : LookupNDDirect  NumberOfTableDimensions=1  Table=gs2_q_f(60:64:end)  DiagnosticForOutOfRangeInput=Error  TableDataTypeStr=fixdt(1,16,15)
  lut_gs1q_58 : LookupNDDirect  NumberOfTableDimensions=1  Table=gs2_q_f(61:64:end)  DiagnosticForOutOfRangeInput=Error  TableDataTypeStr=fixdt(1,16,15)
  lut_gs1q_59 : LookupNDDirect  NumberOfTableDimensions=1  Table=gs2_q_f(62:64:end)  DiagnosticForOutOfRangeInput=Error  TableDataTypeStr=fixdt(1,16,15)
  lut_gs1q_6 : LookupNDDirect  NumberOfTableDimensions=1  Table=gs2_q_f(14:64:end)  DiagnosticForOutOfRangeInput=Error  TableDataTypeStr=fixdt(1,16,15)
  lut_gs1q_60 : LookupNDDirect  NumberOfTableDimensions=1  Table=gs2_q_f(63:64:end)  DiagnosticForOutOfRangeInput=Error  TableDataTypeStr=fixdt(1,16,15)
  lut_gs1q_61 : LookupNDDirect  NumberOfTableDimensions=1  Table=gs2_q_f(64:64:end)  DiagnosticForOutOfRangeInput=Error  TableDataTypeStr=fixdt(1,16,15)
  lut_gs1q_62 : LookupNDDirect  NumberOfTableDimensions=1  Table=gs2_q_f(7:64:end)  DiagnosticForOutOfRangeInput=Error  TableDataTypeStr=fixdt(1,16,15)
  lut_gs1q_63 : LookupNDDirect  NumberOfTableDimensions=1  Table=gs2_q_f(8:64:end)  DiagnosticForOutOfRangeInput=Error  TableDataTypeStr=fixdt(1,16,15)
  lut_gs1q_64 : LookupNDDirect  NumberOfTableDimensions=1  Table=gs2_q_f(9:64:end)  DiagnosticForOutOfRangeInput=Error  TableDataTypeStr=fixdt(1,16,15)
  lut_gs1q_7 : LookupNDDirect  NumberOfTableDimensions=1  Table=gs2_q_f(15:64:end)  DiagnosticForOutOfRangeInput=Error  TableDataTypeStr=fixdt(1,16,15)
  lut_gs1q_8 : LookupNDDirect  NumberOfTableDimensions=1  Table=gs2_q_f(16:64:end)  DiagnosticForOutOfRangeInput=Error  TableDataTypeStr=fixdt(1,16,15)
  lut_gs1q_9 : LookupNDDirect  NumberOfTableDimensions=1  Table=gs2_q_f(17:64:end)  DiagnosticForOutOfRangeInput=Error  TableDataTypeStr=fixdt(1,16,15)
  gs1_i : Outport
  gs1_q : Outport  Port=2
  wires:
  addr/1 -> Data Type Conversion/1
  Delay/1 -> gs1_i/1
  Delay1/1 -> gs1_q/1
  lut_gs1i_1/1 -> Vector Concatenate/64
  lut_gs1i_2/1 -> Vector Concatenate/63
  lut_gs1i_3/1 -> Vector Concatenate/62
  lut_gs1i_4/1 -> Vector Concatenate/61
  lut_gs1i_5/1 -> Vector Concatenate/60
  lut_gs1i_6/1 -> Vector Concatenate/59
  lut_gs1i_7/1 -> Vector Concatenate/58
  lut_gs1i_8/1 -> Vector Concatenate/57
  lut_gs1i_9/1 -> Vector Concatenate/56
  lut_gs1i_10/1 -> Vector Concatenate/55
  lut_gs1i_11/1 -> Vector Concatenate/54
  lut_gs1i_12/1 -> Vector Concatenate/53
  lut_gs1i_13/1 -> Vector Concatenate/52
  lut_gs1i_14/1 -> Vector Concatenate/51
  lut_gs1i_15/1 -> Vector Concatenate/50
  lut_gs1i_16/1 -> Vector Concatenate/49
  lut_gs1i_17/1 -> Vector Concatenate/48
  lut_gs1i_18/1 -> Vector Concatenate/47
  lut_gs1i_19/1 -> Vector Concatenate/46
  lut_gs1i_20/1 -> Vector Concatenate/45
  lut_gs1i_21/1 -> Vector Concatenate/44
  lut_gs1i_22/1 -> Vector Concatenate/43
  lut_gs1i_23/1 -> Vector Concatenate/42
  lut_gs1i_24/1 -> Vector Concatenate/41
  lut_gs1i_25/1 -> Vector Concatenate/40
  lut_gs1i_26/1 -> Vector Concatenate/39
  lut_gs1i_27/1 -> Vector Concatenate/38
  lut_gs1i_28/1 -> Vector Concatenate/37
  lut_gs1i_29/1 -> Vector Concatenate/36
  lut_gs1i_30/1 -> Vector Concatenate/35
  lut_gs1i_31/1 -> Vector Concatenate/34
  lut_gs1i_32/1 -> Vector Concatenate/33
  lut_gs1i_33/1 -> Vector Concatenate/32
  lut_gs1i_34/1 -> Vector Concatenate/31
  lut_gs1i_35/1 -> Vector Concatenate/30
  lut_gs1i_36/1 -> Vector Concatenate/29
  lut_gs1i_37/1 -> Vector Concatenate/28
  lut_gs1i_38/1 -> Vector Concatenate/27
  lut_gs1i_39/1 -> Vector Concatenate/26
  lut_gs1i_40/1 -> Vector Concatenate/25
  lut_gs1i_41/1 -> Vector Concatenate/24
  lut_gs1i_42/1 -> Vector Concatenate/23
  lut_gs1i_43/1 -> Vector Concatenate/22
  lut_gs1i_44/1 -> Vector Concatenate/21
  lut_gs1i_45/1 -> Vector Concatenate/20
  lut_gs1i_46/1 -> Vector Concatenate/19
  lut_gs1i_47/1 -> Vector Concatenate/18
  lut_gs1i_48/1 -> Vector Concatenate/17
  lut_gs1i_49/1 -> Vector Concatenate/16
  lut_gs1i_50/1 -> Vector Concatenate/15
  lut_gs1i_51/1 -> Vector Concatenate/14
  lut_gs1i_52/1 -> Vector Concatenate/13
  lut_gs1i_53/1 -> Vector Concatenate/12
  lut_gs1i_54/1 -> Vector Concatenate/11
  lut_gs1i_55/1 -> Vector Concatenate/10
  lut_gs1i_56/1 -> Vector Concatenate/9
  lut_gs1i_57/1 -> Vector Concatenate/8
  lut_gs1i_58/1 -> Vector Concatenate/7
  lut_gs1i_59/1 -> Vector Concatenate/6
  lut_gs1i_60/1 -> Vector Concatenate/5
  lut_gs1i_61/1 -> Vector Concatenate/4
  lut_gs1i_62/1 -> Vector Concatenate/3
  lut_gs1i_63/1 -> Vector Concatenate/2
  lut_gs1i_64/1 -> Vector Concatenate/1
  Vector Concatenate/1 -> Delay/1
  lut_gs1q_17/1 -> Vector Concatenate1/41
  lut_gs1q_55/1 -> Vector Concatenate1/6
  lut_gs1q_44/1 -> Vector Concatenate1/16
  lut_gs1q_16/1 -> Vector Concatenate1/42
  lut_gs1q_51/1 -> Vector Concatenate1/10
  lut_gs1q_54/1 -> Vector Concatenate1/7
  lut_gs1q_18/1 -> Vector Concatenate1/40
  lut_gs1q_42/1 -> Vector Concatenate1/18
  lut_gs1q_22/1 -> Vector Concatenate1/36
  lut_gs1q_64/1 -> Vector Concatenate1/56
  lut_gs1q_63/1 -> Vector Concatenate1/57
  lut_gs1q_60/1 -> Vector Concatenate1/2
  lut_gs1q_2/1 -> Vector Concatenate1/55
  lut_gs1q_27/1 -> Vector Concatenate1/32
  lut_gs1q_11/1 -> Vector Concatenate1/46
  lut_gs1q_43/1 -> Vector Concatenate1/17
  lut_gs1q_30/1 -> Vector Concatenate1/29
  lut_gs1q_19/1 -> Vector Concatenate1/39
  lut_gs1q_5/1 -> Vector Concatenate1/52
  lut_gs1q_23/1 -> Vector Concatenate1/62
  lut_gs1q_38/1 -> Vector Concatenate1/22
  lut_gs1q_53/1 -> Vector Concatenate1/8
  lut_gs1q_35/1 -> Vector Concatenate1/25
  lut_gs1q_1/1 -> Vector Concatenate1/64
  lut_gs1q_10/1 -> Vector Concatenate1/47
  lut_gs1q_7/1 -> Vector Concatenate1/50
  lut_gs1q_24/1 -> Vector Concatenate1/35
  lut_gs1q_9/1 -> Vector Concatenate1/48
  lut_gs1q_13/1 -> Vector Concatenate1/45
  lut_gs1q_32/1 -> Vector Concatenate1/27
  lut_gs1q_37/1 -> Vector Concatenate1/23
  lut_gs1q_58/1 -> Vector Concatenate1/4
  lut_gs1q_6/1 -> Vector Concatenate1/51
  lut_gs1q_52/1 -> Vector Concatenate1/9
  lut_gs1q_57/1 -> Vector Concatenate1/5
  lut_gs1q_33/1 -> Vector Concatenate1/26
  lut_gs1q_15/1 -> Vector Concatenate1/43
  lut_gs1q_31/1 -> Vector Concatenate1/28
  lut_gs1q_25/1 -> Vector Concatenate1/34
  lut_gs1q_39/1 -> Vector Concatenate1/21
  lut_gs1q_28/1 -> Vector Concatenate1/31
  lut_gs1q_49/1 -> Vector Concatenate1/12
  lut_gs1q_26/1 -> Vector Concatenate1/33
  lut_gs1q_59/1 -> Vector Concatenate1/3
  lut_gs1q_34/1 -> Vector Concatenate1/61
  lut_gs1q_8/1 -> Vector Concatenate1/49
  lut_gs1q_50/1 -> Vector Concatenate1/11
  lut_gs1q_4/1 -> Vector Concatenate1/53
  lut_gs1q_46/1 -> Vector Concatenate1/15
  Data Type Conversion/1 -> lut_gs1q_34/1, lut_gs1q_63/1, lut_gs1q_62/1, lut_gs1q_56/1, lut_gs1q_45/1, lut_gs1q_23/1, lut_gs1q_12/1, lut_gs1q_54/1, lut_gs1q_55/1, lut_gs1q_57/1, lut_gs1q_59/1, lut_gs1q_60/1, lut_gs1q_61/1, lut_gs1q_58/1, lut_gs1q_53/1, lut_gs1q_46/1, lut_gs1q_47/1, lut_gs1q_48/1, lut_gs1q_49/1, lut_gs1q_50/1, lut_gs1q_51/1, lut_gs1q_52/1, lut_gs1q_44/1, lut_gs1q_37/1, lut_gs1q_38/1, lut_gs1q_39/1, lut_gs1q_40/1, lut_gs1q_41/1, lut_gs1q_43/1, lut_gs1q_42/1, lut_gs1q_36/1, lut_gs1q_28/1, lut_gs1q_31/1, lut_gs1q_32/1, lut_gs1q_33/1, lut_gs1q_35/1, lut_gs1q_30/1, lut_gs1q_29/1, lut_gs1q_27/1, lut_gs1q_19/1, lut_gs1q_21/1, lut_gs1q_22/1, lut_gs1q_24/1, lut_gs1q_26/1, lut_gs1q_25/1, lut_gs1q_20/1, lut_gs1q_18/1, lut_gs1q_10/1, lut_gs1q_14/1, lut_gs1q_16/1, lut_gs1q_17/1, lut_gs1q_15/1, lut_gs1q_13/1, lut_gs1q_11/1, lut_gs1q_9/1, lut_gs1q_8/1, lut_gs1q_7/1, lut_gs1q_6/1, lut_gs1q_5/1, lut_gs1q_4/1, lut_gs1q_3/1, lut_gs1q_2/1, lut_gs1q_64/1, lut_gs1q_1/1, lut_gs1i_4/1, lut_gs1i_8/1, lut_gs1i_7/1, lut_gs1i_6/1, lut_gs1i_5/1, lut_gs1i_3/1, lut_gs1i_2/1, lut_gs1i_58/1, lut_gs1i_59/1, lut_gs1i_60/1, lut_gs1i_62/1, lut_gs1i_63/1, lut_gs1i_64/1, lut_gs1i_61/1, lut_gs1i_57/1, lut_gs1i_50/1, lut_gs1i_51/1, lut_gs1i_52/1, lut_gs1i_53/1, lut_gs1i_54/1, lut_gs1i_55/1, lut_gs1i_56/1, lut_gs1i_49/1, lut_gs1i_42/1, lut_gs1i_43/1, lut_gs1i_44/1, lut_gs1i_45/1, lut_gs1i_46/1, lut_gs1i_48/1, lut_gs1i_47/1, lut_gs1i_41/1, lut_gs1i_34/1, lut_gs1i_37/1, lut_gs1i_38/1, lut_gs1i_39/1, lut_gs1i_40/1, lut_gs1i_36/1, lut_gs1i_35/1, lut_gs1i_33/1, lut_gs1i_26/1, lut_gs1i_28/1, lut_gs1i_29/1, lut_gs1i_30/1, lut_gs1i_32/1, lut_gs1i_31/1, lut_gs1i_27/1, lut_gs1i_25/1, lut_gs1i_18/1, lut_gs1i_21/1, lut_gs1i_23/1, lut_gs1i_24/1, lut_gs1i_22/1, lut_gs1i_20/1, lut_gs1i_19/1, lut_gs1i_17/1, lut_gs1i_16/1, lut_gs1i_15/1, lut_gs1i_14/1, lut_gs1i_13/1, lut_gs1i_12/1, lut_gs1i_11/1, lut_gs1i_10/1, lut_gs1i_9/1, lut_gs1i_1/1
  lut_gs1q_56/1 -> Vector Concatenate1/59
  lut_gs1q_14/1 -> Vector Concatenate1/44
  lut_gs1q_41/1 -> Vector Concatenate1/19
  lut_gs1q_21/1 -> Vector Concatenate1/37
  lut_gs1q_20/1 -> Vector Concatenate1/38
  lut_gs1q_40/1 -> Vector Concatenate1/20
  Vector Concatenate1/1 -> Delay1/1
  lut_gs1q_3/1 -> Vector Concatenate1/54
  lut_gs1q_48/1 -> Vector Concatenate1/13
  lut_gs1q_62/1 -> Vector Concatenate1/58
  lut_gs1q_45/1 -> Vector Concatenate1/60
  lut_gs1q_12/1 -> Vector Concatenate1/63
  lut_gs1q_29/1 -> Vector Concatenate1/30
  lut_gs1q_47/1 -> Vector Concatenate1/14
  lut_gs1q_61/1 -> Vector Concatenate1/1
  lut_gs1q_36/1 -> Vector Concatenate1/24

== system ZynqBF_2tx_fpga/channel_estimator/peakdetect_ch2/correlator2/rx_ram_i ==
  i : Inport  Partition=on  PartitionDimension=1  PartitionWidth=1  PartitionOffset=0
  wdata : Inport  Port=2
  waddr : Inport  Port=3
  we : Inport  Port=4
  raddr : Inport  Port=5
  shift : Inport  Port=6
  Constant : Constant  OutDataTypeStr=fixdt(0,1,0)  SampleTime=-1
  Constant1 : Constant  OutDataTypeStr=fixdt(0,1,0)  SampleTime=-1
  For Each : ForEach  DisableCoverage=on  IndexMode=One-based
  Relational Operator : RelationalOperator  Operator=<  OutDataTypeStr=boolean  RndMeth=Nearest
  Simple Dual Port RAM : hdlsllib/HDL RAMs/Simple Dual Port RAM  ram_size=9
      settings: SourceProductName=HDL Coder  SourceProductBaseCode=HD
  Sum : Sum  Inputs=|++  OutDataTypeStr=fixdt(0,9,0)
  Sum1 : Sum  Inputs=|++  OutDataTypeStr=fixdt(0,9,0)
  Switch : Switch  Criteria=u2 ~= 0
  get_bit : MATLAB Function  TreatAsAtomicUnit=on
  dout : Outport  ConcatenationDimension=1
  probe : Outport  Port=2  ConcatenationDimension=1
  wires:
  Sum1/1 -> get_bit/2(ind)
  i/1 -> Sum1/1, Relational Operator/1
  Constant1/1 -> Sum1/2
  Switch/1 -> probe/1, Simple Dual Port RAM/4
  Relational Operator/1 -> Switch/2
  Sum/1 -> Switch/1
  Constant/1 -> Sum/1
  raddr/1 -> Switch/3, Sum/2
  shift/1 -> Relational Operator/2
  Simple Dual Port RAM/1 -> dout/1
  get_bit/1(y) -> Simple Dual Port RAM/3
  we/1 -> get_bit/1(u)
  waddr/1 -> Simple Dual Port RAM/2
  wdata/1 -> Simple Dual Port RAM/1

== system ZynqBF_2tx_fpga/channel_estimator/peakdetect_ch2/correlator2/rx_ram_q ==
  i : Inport  Partition=on  PartitionDimension=1  PartitionWidth=1  PartitionOffset=0
  wdata : Inport  Port=2
  waddr : Inport  Port=3
  we : Inport  Port=4
  raddr : Inport  Port=5
  shift : Inport  Port=6
  Constant : Constant  OutDataTypeStr=fixdt(0,1,0)  SampleTime=-1
  Constant1 : Constant  OutDataTypeStr=fixdt(0,1,0)  SampleTime=-1
  For Each : ForEach  DisableCoverage=on  IndexMode=One-based
  Relational Operator : RelationalOperator  Operator=<  OutDataTypeStr=boolean  RndMeth=Nearest
  Simple Dual Port RAM : hdlsllib/HDL RAMs/Simple Dual Port RAM  ram_size=9
      settings: SourceProductName=HDL Coder  SourceProductBaseCode=HD
  Sum : Sum  Inputs=|++  OutDataTypeStr=fixdt(0,9,0)
  Sum1 : Sum  Inputs=|++  OutDataTypeStr=fixdt(0,9,0)
  Switch : Switch  Criteria=u2 ~= 0
  get_bit : MATLAB Function  TreatAsAtomicUnit=on
  dout : Outport  ConcatenationDimension=1
  probe : Outport  Port=2  ConcatenationDimension=1
  wires:
  Sum1/1 -> get_bit/2(ind)
  i/1 -> Sum1/1, Relational Operator/1
  Constant1/1 -> Sum1/2
  Switch/1 -> probe/1, Simple Dual Port RAM/4
  Relational Operator/1 -> Switch/2
  Sum/1 -> Switch/1
  Constant/1 -> Sum/1
  raddr/1 -> Switch/3, Sum/2
  shift/1 -> Relational Operator/2
  Simple Dual Port RAM/1 -> dout/1
  get_bit/1(y) -> Simple Dual Port RAM/3
  we/1 -> get_bit/1(u)
  waddr/1 -> Simple Dual Port RAM/2
  wdata/1 -> Simple Dual Port RAM/1

== system ZynqBF_2tx_fpga/channel_estimator/peakdetect_ch2/correlator2/sum_elements_i ==
  din : Inport  Partition=on  PartitionDimension=1  PartitionWidth=8  PartitionOffset=0
  start : Inport  Port=2
  Add : Sum  OutDataTypeStr=fixdt(1,32,16)
  Compare To Constant1 : simulink/Logic and Bit Operations/Compare To Constant  relop===  const=7  OutDataTypeStr=boolean
  Compare To Constant2 : simulink/Logic and Bit Operations/Compare To Constant  relop===  const=1  OutDataTypeStr=boolean
  Constant : Constant  Value=0  OutDataTypeStr=fixdt(1,32,16)  SampleTime=-1
  Constant1 : Constant  Value=0  OutDataTypeStr=fixdt(1,16,15)  SampleTime=-1
  Data Type Conversion : DataTypeConversion  OutDataTypeStr=uint8
  Delay1 : Delay  DelayLength=1
  For Each : ForEach  DisableCoverage=on  IndexMode=One-based
  HDL Counter : hdlsllib/Sources/HDL Counter  CountType=Free running  CountInit=0  CountStep=1  CountMax=64  CountFromType=Initial value  CountFrom=0  CountResetPort=on  CountLoadPort=off  CountEnbPort=on  CountDirPort=off  CountDataType=Unsigned  CountWordLen=3  CountFracLen=0  CountSampTime=1
      settings: SourceProductBaseCode=HD
  HDL Counter1 : hdlsllib/Sources/HDL Counter  CountType=Free running  CountInit=0  CountStep=1  CountMax=64  CountFromType=Initial value  CountFrom=0  CountResetPort=off  CountLoadPort=off  CountEnbPort=on  CountDirPort=off  CountDataType=Unsigned  CountWordLen=1  CountFracLen=0  CountSampTime=1
      settings: SourceProductBaseCode=HD
  Logical Operator : Logic  Operator=OR  IconShape=distinctive  AllPortsSameDT=off  OutDataTypeStr=boolean
  Selector : Selector  IndexMode=Zero-based  InputPortWidth=8  IndexOptions=Starting index (port)  Indices=[1 3]  OutputSizes=1
  Switch : Switch  Criteria=u2 ~= 0
  Switch1 : Switch  Criteria=u2 ~= 0
  dout : Outport  ConcatenationDimension=1
  vout : Outport  Port=2  ConcatenationDimension=1
  wires:
  HDL Counter/1 -> Data Type Conversion/1, Compare To Constant1/1
  Logical Operator/1 -> HDL Counter1/1
  Data Type Conversion/1 -> Selector/2
  din/1 -> Selector/1
  Selector/1 -> Switch1/1
  HDL Counter1/1 -> Compare To Constant2/1
  Constant1/1 -> Switch1/3
  Switch1/1 -> Add/1
  Constant/1 -> Switch/1
  Switch/1 -> Add/2
  Delay1/1 -> Switch/3
  Compare To Constant1/1 -> vout/1, Logical Operator/2
  Compare To Constant2/1 -> HDL Counter/2, Switch1/2
  Add/1 -> dout/1, Delay1/1
  start/1 -> HDL Counter/1, Switch/2, Logical Operator/1

== system ZynqBF_2tx_fpga/channel_estimator/peakdetect_ch2/correlator2/sum_elements_q ==
  din : Inport  Partition=on  PartitionDimension=1  PartitionWidth=8  PartitionOffset=0
  start : Inport  Port=2
  Add : Sum  OutDataTypeStr=fixdt(1,32,16)
  Compare To Constant1 : simulink/Logic and Bit Operations/Compare To Constant  relop===  const=7  OutDataTypeStr=boolean
  Compare To Constant2 : simulink/Logic and Bit Operations/Compare To Constant  relop===  const=1  OutDataTypeStr=boolean
  Constant : Constant  Value=0  OutDataTypeStr=fixdt(1,32,16)  SampleTime=-1
  Constant1 : Constant  Value=0  OutDataTypeStr=fixdt(1,16,15)  SampleTime=-1
  Data Type Conversion : DataTypeConversion  OutDataTypeStr=uint8
  Delay1 : Delay  DelayLength=1
  For Each : ForEach  DisableCoverage=on  IndexMode=One-based
  HDL Counter : hdlsllib/Sources/HDL Counter  CountType=Free running  CountInit=0  CountStep=1  CountMax=64  CountFromType=Initial value  CountFrom=0  CountResetPort=on  CountLoadPort=off  CountEnbPort=on  CountDirPort=off  CountDataType=Unsigned  CountWordLen=3  CountFracLen=0  CountSampTime=1
      settings: SourceProductBaseCode=HD
  HDL Counter1 : hdlsllib/Sources/HDL Counter  CountType=Free running  CountInit=0  CountStep=1  CountMax=64  CountFromType=Initial value  CountFrom=0  CountResetPort=off  CountLoadPort=off  CountEnbPort=on  CountDirPort=off  CountDataType=Unsigned  CountWordLen=1  CountFracLen=0  CountSampTime=1
      settings: SourceProductBaseCode=HD
  Logical Operator : Logic  Operator=OR  IconShape=distinctive  AllPortsSameDT=off  OutDataTypeStr=boolean
  Selector : Selector  IndexMode=Zero-based  InputPortWidth=8  IndexOptions=Starting index (port)  Indices=[1 3]  OutputSizes=1
  Switch : Switch  Criteria=u2 ~= 0
  Switch1 : Switch  Criteria=u2 ~= 0
  dout : Outport  ConcatenationDimension=1
  vout : Outport  Port=2  ConcatenationDimension=1
  wires:
  HDL Counter/1 -> Data Type Conversion/1, Compare To Constant1/1
  Logical Operator/1 -> HDL Counter1/1
  Data Type Conversion/1 -> Selector/2
  din/1 -> Selector/1
  Selector/1 -> Switch1/1
  HDL Counter1/1 -> Compare To Constant2/1
  Constant1/1 -> Switch1/3
  Switch1/1 -> Add/1
  Constant/1 -> Switch/1
  Switch/1 -> Add/2
  Delay1/1 -> Switch/3
  Compare To Constant1/1 -> vout/1, Logical Operator/2
  Compare To Constant2/1 -> HDL Counter/2, Switch1/2
  Add/1 -> dout/1, Delay1/1
  start/1 -> HDL Counter/1, Switch/2, Logical Operator/1
